simulink model "temperature"  (R2013b)
settings: Solver=ode3  SolverMode=SingleTasking  StartTime=0.0  StopTime=400.0  RelTol=1e-3
libraries: arduino_io_lib x4
settings Model: ExtModeTrigDuration=2  Creator=gcampa  LastModifiedBy=richard.hill
settings OptimizationCC: OptimizeModelRefInitCode=on  LifeSpan=1
settings DebuggingCC: SolverPrmCheckMsg=none
settings HardwareCC: ProdBitPerInt=16  ProdBitPerPointer=8  ProdIntDivRoundTo=Zero  ProdEndianess=LittleEndian  ProdWordSize=8  ProdHWDeviceType=Atmel->AVR
settings RTWCC: SystemTargetFile=realtime.tlc  GenerateMakefile=off  TemplateMakefile=realtime.tmf  Description=Run on Target Hardware  RTWVerbose=off  ProcessScript=realtime_make_rtw_hook
settings STFCustomTargetCC: TargetLibSuffix=.a  GenerateSampleERTMain=on  ERTCustomFileBanners=on  SupportNonInlinedSFcns=off  SupportVariableSizeSignals=on  MATLABClassNameForMDSCustomization=Simulink.SoftwareTarget.ERTCustomization  GRTInterface=off  SystemTargetFile=realtime.tlc
settings ERTTargetCC: CodeReplacementLibrary=ANSI_C  GenerateSampleERTMain=on  ParMdlRefBuildCompliant=off  CompOptLevelCompliant=off  ConcurrentExecutionCompliant=off  CombineOutputUpdateFcns=off  ERTFirstTimeCompliant=off  SupportContinuousTime=on  SupportVariableSizeSignals=on  ModelStepFunctionPrototypeControlCompliant=off  CPPClassGenCompliant=off  ExtModeTransport=3  ExtModeMexFile=ext_serial_win32_comm  ExtModeMexArgs=0 1 9600  InlinedParameterPlacement=NonHierarchical  ERTSrcFileBannerTemplate=realtime_code_template.cgt  ERTHdrFileBannerTemplate=realtime_code_template.cgt  ERTDataSrcFileTemplate=realtime_code_template.cgt  ERTDataHdrFileTemplate=realtime_code_template.cgt  ERTCustomFileTemplate=realtime_file_process.tlc

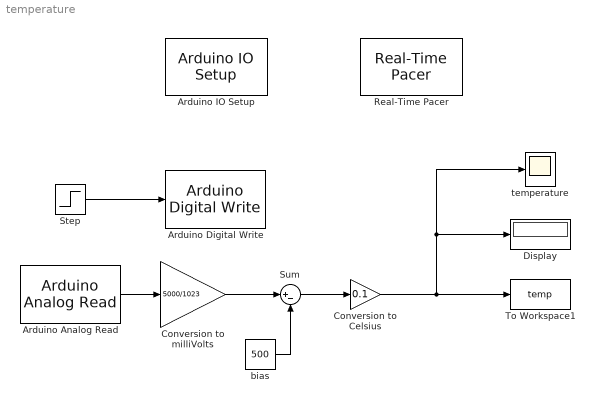
== system temperature ==
  Arduino Analog Read : arduino_io_lib/Arduino Analog Read  arduinoVar=Temporary arduino variable: Arduino1  arduinoPin=0  T=0.1
  Arduino Digital Write : arduino_io_lib/Arduino Digital Write  arduinoVar=Temporary arduino variable: Arduino1  arduinoPin=9  T=0.1
  Arduino IO Setup : arduino_io_lib/Arduino IO Setup  Priority=3  arduinoVar=Temporary arduino variable: Arduino1  workspaceVarName=b  comPort=COM3
  Conversion to Celsius : Gain  Gain=0.1
  Conversion to milliVolts : Gain  Gain=5000/1023
  Display : Display
  Real-Time Pacer : arduino_io_lib/Real-Time Pacer  simTimePerRealTime=1
  Step : Step  Time=10  SampleTime=0
  Sum : Sum  Inputs=|+-
  To Workspace1 : ToWorkspace  VariableName=temp  SampleTime=-1  SaveFormat=Timeseries
  bias : Constant  Value=500
  temperature : Scope
      settings: YMin=15  YMax=120
  wires:
  Arduino Analog Read/1 -> Conversion to milliVolts/1
  Conversion to milliVolts/1 -> Sum/1
  Step/1 -> Arduino Digital Write/1
  Sum/1 -> Conversion to Celsius/1
  Conversion to Celsius/1 -> temperature/1, Display/1, To Workspace1/1
  bias/1 -> Sum/2
